simulink model "Chirp"  (R2024b)
settings: Solver=FixedStepAuto  StartTime=0.0  StopTime=inf  RelTol=1e-3  EnableMultiTasking=on
undefined symbols (not defined in the file or in its folder): dspblkCoreblockFVToolHelper, gcbh
libraries: px4Peripheralslib x1, slpidlib x1, px4uORBlib x1, sharedtransform x1, dspsrcs4 x1, simulink x1, simulink_extras x1
settings Model: SimulationMode=external  ExtModeTrigDuration=10  Creator=luker  LastModifiedBy=Adrial Naidoo
settings SolverCC: ConcurrentTasks=on  PositivePriorityOrder=on  AutoInsertRateTranBlk=on
settings OptimizationCC: EnhancedBackFolding=on  PassReuseOutputArgsAs=Individual arguments  ZeroExternalMemoryAtStartup=off  ZeroInternalMemoryAtStartup=off  MaxStackSize=64  OptimizeBlockOrder=speed  DifferentSizesBufferReuse=on  EfficientTunableParamExpr=on
settings DebuggingCC: ParameterTunabilityLossMsg=error
settings HardwareCC: ProdBitPerPointer=32  ProdBitPerSizeT=32  ProdBitPerPtrDiffT=32  ProdLargestAtomicInteger=Long  ProdLargestAtomicFloat=Double  ProdWordSize=32  ProdLongLongMode=on  ProdHWDeviceType=ARM Compatible->ARM Cortex
settings SFSimCC: MATLABDynamicMemAlloc=off  SimTargetLang=C++
settings RTWCC: Description=Embedded Coder  SystemTargetFile=ert.tlc  HardwareBoard=PX4 Pixhawk Series  TLCOptions="-aInlineSetEventsForThisBaseRateFcn=TLC_FALSE -aSuppressMultiTaskScheduler=TLC_FALSE  -aRateBasedStepFcn=0"  TemplateMakefile=ert_default_tmf  Toolchain=GNU Tools for PX4 Autopilots  TargetLang=C++
settings CodeAppCC: ForceParamTrailComments=on  IgnoreCustomStorageClasses=off  OperatorAnnotations=on  SimulinkDataObjDesc=on  SFDataObjDesc=on  InsertBlockDesc=on
settings ERTTargetCC: SupportContinuousTime=on  ExtModeTransport=3  ExtModeStaticAlloc=on  ExtModeStaticAllocSize=1024  ExtModeMexFile=ext_xcp  ExtModeIntrfLevel=Level2 - Open  InlinedParameterPlacement=Hierarchical  RTWCAPISignals=on  RTWCAPIParams=on  RTWCAPIStates=on

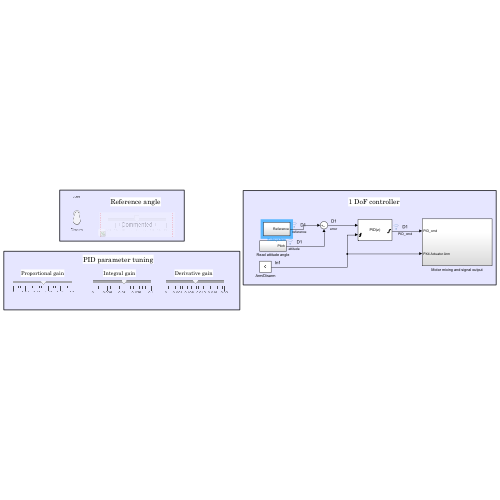
[thumbnail: Simulink's stored preview of the top-level diagram]
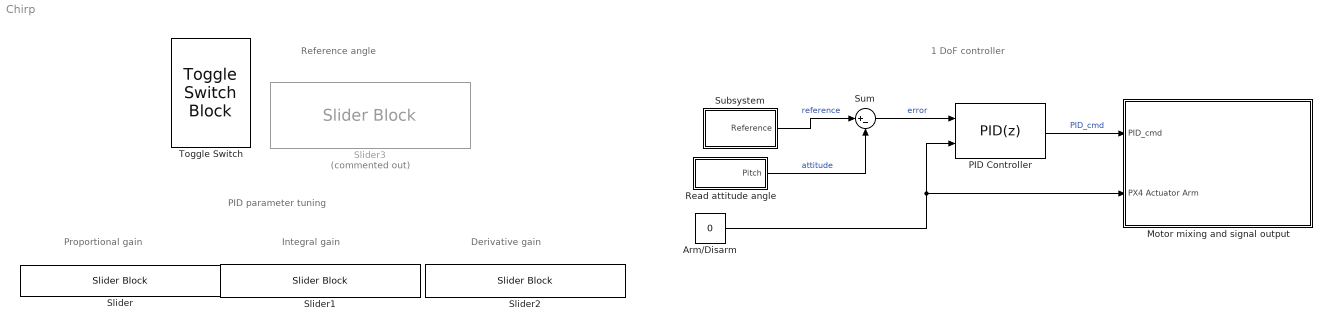
== system Chirp ==
  note: Proportional gain
  note: Reference angle
  note: PID parameter tuning
  note: Integral gain
  note: Derivative gain
  note: 1 DoF controller
  Arm/Disarm : Constant  Value=0
  Motor mixing and signal output : Subsystem
  PID Controller : slpidlib/PID Controller  Controller=PID  Form=Parallel  TimeDomain=Discrete-time  UseExternalTs=off  SampleTime=0.007  IntegratorMethod=Forward Euler  FilterMethod=Forward Euler  ControllerParametersSource=internal  P=0.1027863777089783  I=0.05424823410696267  UseKiTs=off  D=0.01003095975232198  UseExternalDerivativeSource=off  N=60  UseFilter=on  TunerSelectOption=Transfer Function Based (PID Tuner App)  InitialConditionSource=internal  InitialConditionForIntegrator=0  InitialConditionForFilter=0  DifferentiatorICPrevScaledInput=0  ExternalReset=rising  TrackingMode=off  Kt=1  LimitOutput=on  SatLimitsSource=internal  UpperSaturationLimit=0.5  LowerSaturationLimit=-0.5  LinearizeAsGain=off  AntiWindupMode=back-calculation  Kb=100  LimitIntegrator=on  UpperIntegratorSaturationLimit=0.08  LowerIntegratorSaturationLimit=-0.08  POutMin=[]  POutMax=[]  IOutMin=[]  IOutMax=[]  DOutMin=[]  DOutMax=[]  NOutMin=[]  NOutMax=[]  SumOutMin=[]  SumOutMax=[]  SaturationOutMin=[]  SaturationOutMax=[]  PParamMin=[]  PParamMax=[]  IParamMin=[]  IParamMax=[]  DParamMin=[]  DParamMax=[]  NParamMin=[]  NParamMax=[]  KbParamMin=[]  KbParamMax=[]  KtParamMin=[]  KtParamMax=[]  KbOutMin=[]  KbOutMax=[]  KtOutMin=[]  KtOutMax=[]  IntegratorOutMin=[]  IntegratorOutMax=[]  FilterOutMin=[]  FilterOutMax=[]  SumI1OutMin=[]  SumI1OutMax=[]  SumI2OutMin=[]  SumI2OutMax=[]  SumI3OutMin=[]  SumI3OutMax=[]  SumI4OutMin=[]  SumI4OutMax=[]  SumDOutMin=[]  SumDOutMax=[]  DifferentiatorOutMin=[]  DifferentiatorOutMax=[]  FilterDiffOutCoefMin=[]  FilterDiffOutCoefMax=[]  ReciprocalOutMin=[]  ReciprocalOutMax=[]  SumDenOutMin=[]  SumDenOutMax=[]  SumNumOutMin=[]  SumNumOutMax=[]  DivideOutMin=[]  DivideOutMax=[]  UdiffTsProdOutMin=[]  UdiffTsProdOutMax=[]  NTsProdOutMin=[]  NTsProdOutMax=[]  UintegralTsProdOutMin=[]  UintegralTsProdOutMax=[]  UngainTsProdOutMin=[]  UngainTsProdOutMax=[]  ClampingZeroOutDataTypeStr=Inherit: Inherit via back propagation  ClampingZeroOutMin=[]  ClampingZeroOutMax=[]  FilterDenConstantOutDataTypeStr=Inherit: Inherit via back propagation  FilterDenConstantOutMin=[]  FilterDenConstantOutMax=[]  PCopyOutDataTypeStr=Inherit: Inherit via back propagation  PCopyOutMin=[]  PCopyOutMax=[]  NCopyOutDataTypeStr=Inherit: Inherit via back propagation  NCopyOutMin=[]  NCopyOutMax=[]  IntegratorContinuousStateAttributes=''  IntegratorStateMustResolveToSignalObject=off  IntegratorRTWStateStorageClass=Auto  FilterContinuousStateAttributes=''  FilterStateMustResolveToSignalObject=off  FilterRTWStateStorageClass=Auto  ParallelPVariant=InternalParameters  IdealPVariant=Disabled  IVariant=InternalParameters  DVariant=InternalParameters  IntegratorVariant=Discrete  SatVariant=Enabled  AWVariant=BackCalculation  PCopyVariant=Disabled  TRVariant=Disabled  FdbkBlocksVariant=Forward  IdealPFdbkVariant=Disabled  SatFdbkVariant=Disabled  DerivativeFilterVariant=ForwardEulerFilter  NVariant=InternalParameters  NCopyVariant=Disabled  FilterICVariant=InternalICsFilter  IntegratorICVariant=InternalICs  ExternalResetVariant=ExternalReset  TRSumVariant=Passthrough  SumFdbkVariant=Disabled  SumVariant=Sum_PID  TsampFilterVariant=InternalTs  TsampNgainVariant=Passthrough  TsampIntegralVariant=Disabled_SignalSpec  ExternalSaturationOutDataTypeStr=Inherit: Same as second input  DerivativeSourceVariant=ErrorSignal  PreIntVariant=InternalPreInt
  Read attitude angle : Subsystem
  Slider : SliderBlock  LabelPosition=Hide  ScaleMax=0.2
  Slider1 : SliderBlock  LabelPosition=Hide  ScaleMax=0.1
  Slider2 : SliderBlock  LabelPosition=Hide  ScaleMax=0.02
  Slider3 : SliderBlock  Commented=on  ScaleMin=-20  ScaleMax=20  TickInterval=5
  Subsystem : Subsystem
  Sum : Sum  Inputs=|+-
  Toggle Switch : ToggleSwitchBlock  LabelPosition=Hide
      settings: Values={{'Disarm', 'Arm'}, [0 1]}
  wires:
  Arm/Disarm/1 -> PID Controller/2, Motor mixing and signal output/2(PX4 Actuator Arm)
  Subsystem/1(Reference) -> Sum/1  "reference"
  Read attitude angle/1(Pitch) -> Sum/2  "attitude"
  Sum/1 -> PID Controller/1  "error"
  PID Controller/1 -> Motor mixing and signal output/1(PID_cmd)  "PID_cmd"

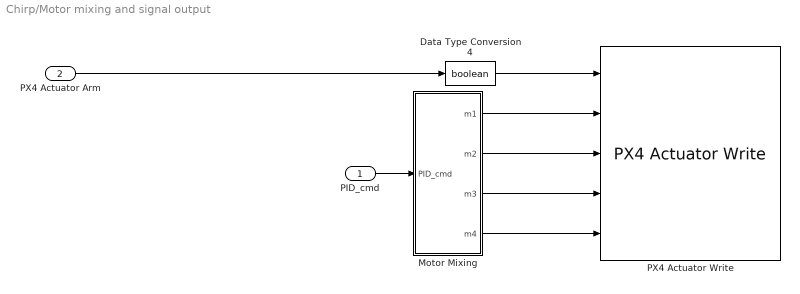
== system Chirp/Motor mixing and signal output ==
  PID_cmd : Inport
  PX4 Actuator Arm : Inport  Port=2
  Data Type Conversion4 : DataTypeConversion  OutDataTypeStr=boolean  SaturateOnIntegerOverflow=off  RndMeth=Floor
  Motor Mixing : Subsystem
  PX4 Actuator Write : px4Peripheralslib/PX4 Actuator Write  Motor1Enable=on  Motor2Enable=on  Motor3Enable=on  Motor4Enable=on  Motor5Enable=off  Motor6Enable=off  Motor7Enable=off  Motor8Enable=off  Motor9Enable=off  Motor10Enable=off  Motor11Enable=off  Motor12Enable=off  IsMotorArray=off  Servo1Enable=off  Servo2Enable=off  Servo3Enable=off  Servo4Enable=off  Servo5Enable=off  Servo6Enable=off  Servo7Enable=off  Servo8Enable=off  IsServoArray=off
      settings: SourceProductName=PX4 Peripheral Blocks
  wires:
  Motor Mixing/2(m2) -> PX4 Actuator Write/3
  Data Type Conversion4/1 -> PX4 Actuator Write/1
  PID_cmd/1 -> Motor Mixing/1(PID_cmd)
  Motor Mixing/3(m3) -> PX4 Actuator Write/4
  Motor Mixing/1(m1) -> PX4 Actuator Write/2
  PX4 Actuator Arm/1 -> Data Type Conversion4/1
  Motor Mixing/4(m4) -> PX4 Actuator Write/5

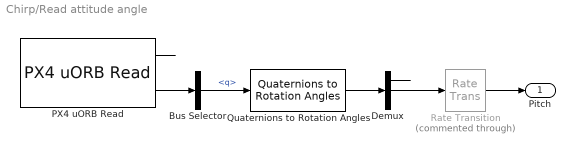
== system Chirp/Read attitude angle ==
  Bus Selector : BusSelector  OutputSignals=q
  Demux : Demux  Outputs=3
  PX4 uORB Read : px4uORBlib/PX4 uORB Read  uORBTopic=VehicleAttitude  selectInstance=vehicle_attitude  SampleTime=-1  BlockingMode=off  BlockTimeout=1e-3
  Quaternions to Rotation Angles : sharedtransform/Quaternions to Rotation Angles  rotationOrder=ZYX  aMode=aMode
  Rate Transition : RateTransition  Commented=through  OutPortSampleTime=0.007
  Pitch : Outport
  wires:
  PX4 uORB Read/1 -> ?
  PX4 uORB Read/2 -> Bus Selector/1
  Quaternions to Rotation Angles/1 -> Demux/1
  Demux/1 -> ?
  Demux/2 -> Rate Transition/1
  Bus Selector/1 -> Quaternions to Rotation Angles/1  "<q>"
  Rate Transition/1 -> Pitch/1

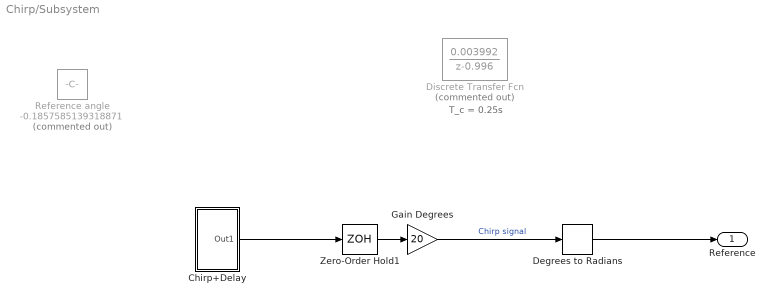
== system Chirp/Subsystem ==
  note: T_c = 0.25s
  Chirp+Delay : Subsystem
  Degrees to Radians : simulink_extras/Transformations/Degrees to Radians
  Discrete Transfer Fcn : DiscreteTransferFcn  Commented=on  LoadFcn=dspblkCoreblockFVToolHelper(gcbh,'load');  Numerator=[0.003992]  Denominator=[1 -0.996]
      settings: CopyFcn=dspblkCoreblockFVToolHelper(gcbh,'copy');  DeleteFcn=dspblkCoreblockFVToolHelper(gcbh,'close');  ModelCloseFcn=dspblkCoreblockFVToolHelper(gcbh,'close');  PreSaveFcn=dspblkCoreblockFVToolHelper(gcbh,'presave');  PostSaveFcn=dspblkCoreblockFVToolHelper(gcbh,'postsave');  CloseFcn=dspblkCoreblockFVToolHelper(gcbh,'close');
  Gain Degrees : Gain  Gain=20
  Reference angle : Constant  Commented=on  Value=-0.1857585139318871
  Zero-Order Hold1 : ZeroOrderHold  SampleTime=0.007
  Reference : Outport
  wires:
  Chirp+Delay/1(Out1) -> Zero-Order Hold1/1
  Gain Degrees/1 -> Degrees to Radians/1  "Chirp signal"
  Degrees to Radians/1 -> Reference/1
  Zero-Order Hold1/1 -> Gain Degrees/1

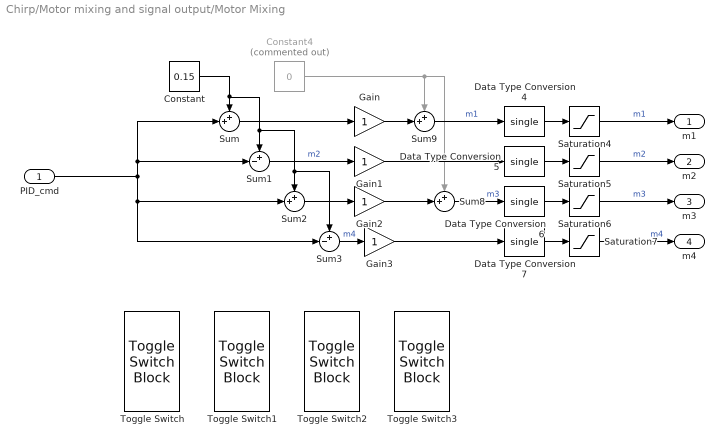
== system Chirp/Motor mixing and signal output/Motor Mixing ==
  PID_cmd : Inport
  Constant : Constant  Value=0.15
  Constant4 : Constant  Commented=on  Value=0
  Data Type Conversion{4..7} (4 alike) : DataTypeConversion  OutDataTypeStr=single  SaturateOnIntegerOverflow=off  RndMeth=Floor
  Gain{,1..3} (4 alike) : Gain
  Saturation{4..7} (4 alike) : Saturate  UpperLimit=1  LowerLimit=0
  Sum{,2,8..9} (4 alike) : Sum  Inputs=++|
  Sum1 : Sum  Inputs=+-|
  Sum3 : Sum  Inputs=+-|
  Toggle Switch{,1..3} (4 alike) : ToggleSwitchBlock
      settings: Values={{'Off', 'On'}, [0 1]}
  m1 : Outport
  m2 : Outport  Port=2
  m3 : Outport  Port=3
  m4 : Outport  Port=4
  wires:
  Constant/1 -> Sum1/1, Sum3/1, Sum2/1, Sum/1
  Sum2/1 -> Gain2/1
  Constant4/1 -> Sum9/1, Sum8/1
  Sum/1 -> Gain/1
  Sum9/1 -> Data Type Conversion4/1  "m1"
  Sum8/1 -> Data Type Conversion6/1  "m3"
  Sum3/1 -> Gain3/1  "m4"
  Sum1/1 -> Gain1/1  "m2"
  Saturation4/1 -> m1/1  "m1"
  Saturation5/1 -> m2/1  "m2"
  Saturation6/1 -> m3/1  "m3"
  Saturation7/1 -> m4/1  "m4"
  Data Type Conversion4/1 -> Saturation4/1
  Data Type Conversion5/1 -> Saturation5/1
  Data Type Conversion6/1 -> Saturation6/1
  Data Type Conversion7/1 -> Saturation7/1
  Gain/1 -> Sum9/2
  Gain1/1 -> Data Type Conversion5/1
  Gain2/1 -> Sum8/2
  Gain3/1 -> Data Type Conversion7/1
  PID_cmd/1 -> Sum2/2, Sum3/2, Sum1/2, Sum/2

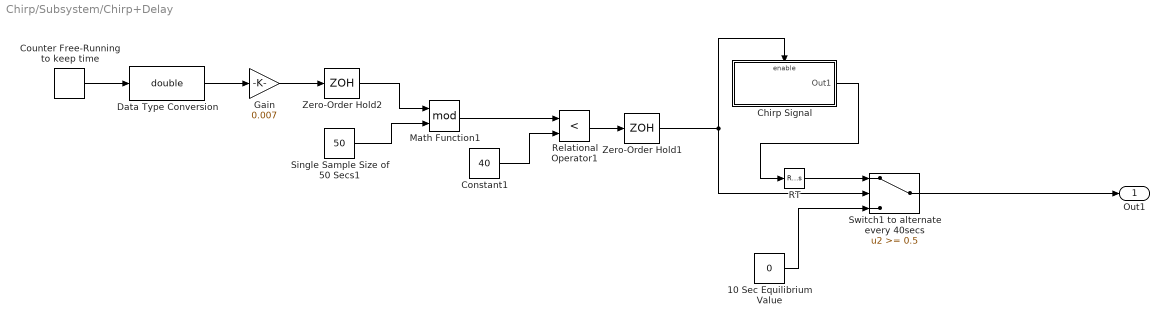
== system Chirp/Subsystem/Chirp+Delay ==
  10 Sec Equilibrium Value : Constant  Value=0  OutDataTypeStr=Inherit: Inherit via back propagation
  Chirp Signal : Subsystem  TreatAsAtomicUnit=on
  Constant1 : Constant  Value=40
  Counter Free-Running to keep time : simulink/Sources/Counter Free-Running  NumBits=16  tsamp=0.007
  Data Type Conversion : DataTypeConversion  OutDataTypeStr=double  SaturateOnIntegerOverflow=off  RndMeth=Floor
  Gain : Gain  Gain=0.007
  Math Function1 : Math  Operator=mod
  RT : RateTransition
  Relational Operator1 : RelationalOperator  Operator=<  OutDataTypeStr=boolean  RndMeth=Simplest  InputSameDT=off
  Single Sample Size of 50 Secs1 : Constant  Value=50
  Switch1 to alternate every 40secs : Switch  Threshold=0.5  SaturateOnIntegerOverflow=off  InputSameDT=off
  Zero-Order Hold1 : ZeroOrderHold  SampleTime=0.007
  Zero-Order Hold2 : ZeroOrderHold  SampleTime=0.007
  Out1 : Outport
  wires:
  Single Sample Size of 50 Secs1/1 -> Math Function1/2
  RT/1 -> Switch1 to alternate every 40secs/1
  10 Sec Equilibrium Value/1 -> Switch1 to alternate every 40secs/3
  Math Function1/1 -> Relational Operator1/1
  Constant1/1 -> Relational Operator1/2
  Switch1 to alternate every 40secs/1 -> Out1/1
  Chirp Signal/1(Out1) -> RT/1
  Relational Operator1/1 -> Zero-Order Hold1/1
  Zero-Order Hold1/1 -> Switch1 to alternate every 40secs/2, Chirp Signal/Enable
  Zero-Order Hold2/1 -> Math Function1/1
  Gain/1 -> Zero-Order Hold2/1
  Counter Free-Running to keep time/1 -> Data Type Conversion/1
  Data Type Conversion/1 -> Gain/1

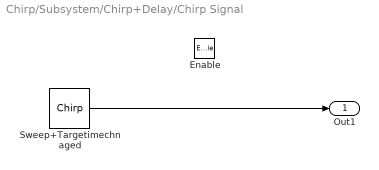
== system Chirp/Subsystem/Chirp+Delay/Chirp Signal ==
  Enable : EnablePort
  Sweep+Targetimechnaged : dspsrcs4/Chirp  sweep=Linear  mode=Bidirectional  f0=0.05  f1=1  t1=5  Tsweep=10  phase=0  Ts=0.007  spf=1  datatype=double  OutputFrames=off
  Out1 : Outport
  wires:
  Sweep+Targetimechnaged/1 -> Out1/1
